simulink model "Vibration modelling"  (R2022b)
settings: Solver=VariableStepAuto  StartTime=0.0  StopTime=10.0  RelTol=1e-3
settings Model: Creator=mluser  LastModifiedBy=mluser
settings DebuggingCC: UnconnectedInputMsg=warning  UnconnectedOutputMsg=warning  UnconnectedLineMsg=warning
settings ModelReferenceCC: EnableRefExpFcnMdlSchedulingChecks=on
settings RTWCC: DLArmComputeVersion=19.05

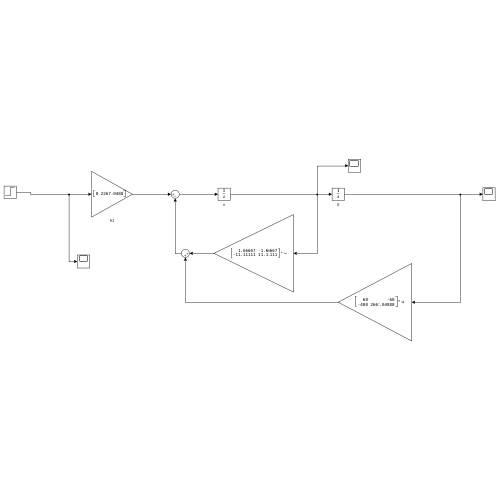
[thumbnail: Simulink's stored preview of the top-level diagram]
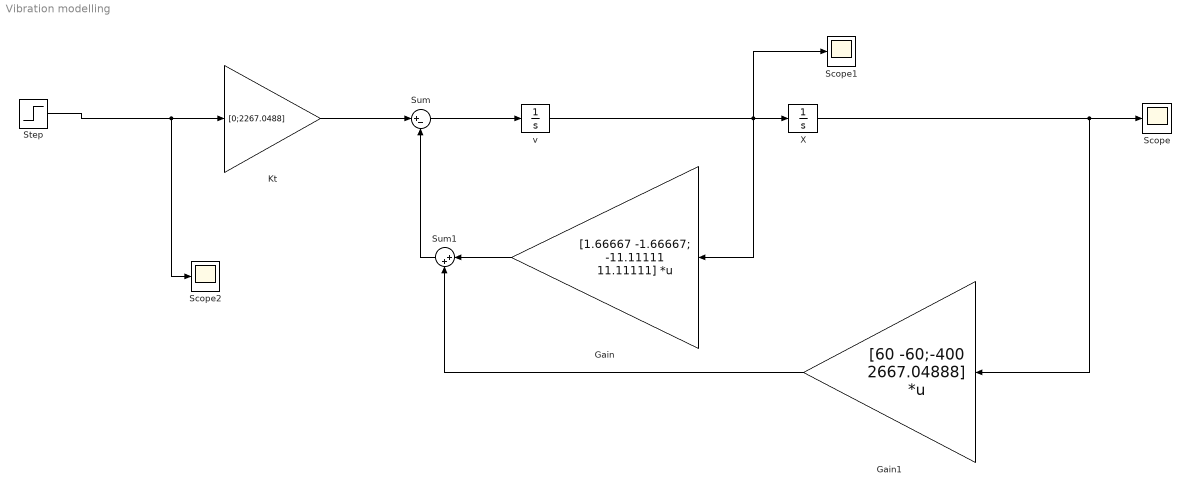
== system Vibration modelling ==
  Gain : Gain  Gain=[1.66667 -1.66667; -11.11111 11.11111]  Multiplication=Matrix(K*u)
  Gain1 : Gain  Gain=[60 -60;-400 2667.04888]  Multiplication=Matrix(K*u)
  Kt : Gain  Gain=[0;2267.0488]
  Scope : Scope
  Scope1 : Scope
  Scope2 : Scope
  Step : Step  SampleTime=0
  Sum : Sum  Inputs=|+-
  Sum1 : Sum  Inputs=|++
  X : Integrator  ContinuousStateAttributes='position'
  v : Integrator  ContinuousStateAttributes='v'
  wires:
  v/1 -> Scope1/1, Gain/1, X/1
  X/1 -> Gain1/1, Scope/1
  Gain/1 -> Sum1/1
  Gain1/1 -> Sum1/2
  Sum1/1 -> Sum/2
  Sum/1 -> v/1
  Kt/1 -> Sum/1
  Step/1 -> Scope2/1, Kt/1
